simulink model "BLDCmotorControl_FOC_R2017b_fixdt"  (R2017b)
settings: Solver=FixedStepDiscrete  StartTime=0  StopTime=0.5  FixedStep=Ts  MaxStep=1e-6  RelTol=1e-6  AbsTol=1e-6  EnableMultiTasking=on
PreLoadFcn:
  | addpath(pwd);
  | addpath(genpath('01_Libraries'));
  | addpath(genpath('02_Figures'));
  | addpath(genpath('03_CreateParamTable'));
InitFcn:
  | init_model;
values from neighbouring files (symbols this model uses):
  a_elecAngle = 60    [init_model.m]
  b_diagEna = 1    [init_model.m]
  b_fieldWeakEna = 0    [init_model.m]
  b_selPhaABCurrMeas = 1    [init_model.m]
  cf_currFilt = 0.12    [init_model.m]
  cf_idKb = 1000 * Ts_ctrl    (= 0.06)    [init_model.m]
  cf_idKi = 100 * Ts_ctrl    (= 0.006)    [init_model.m]
  cf_idKp = 1    [init_model.m]
  cf_iqKb = 1000 * Ts_ctrl    (= 0.06)    [init_model.m]
  cf_iqKi = 100 * Ts_ctrl    (= 0.006)    [init_model.m]
  cf_iqKiLimProt = 40.7 * Ts_ctrl    (= 0.002442)    [init_model.m]
  cf_iqKp = 0.5    [init_model.m]
  cf_iqKpLimProt = 7.2    [init_model.m]
  cf_nKb = 1000 * Ts_ctrl    (= 0.06)    [init_model.m]
  cf_nKi = 20.4 * Ts_ctrl    (= 0.001224)    [init_model.m]
  cf_nKp = 1.18    [init_model.m]
  cf_nKpLimProt = 5    [init_model.m]
  cf_speedCoef = round(f_ctrl * a_mechAngle * (pi/180) * (30/pi))    [init_model.m]
  CTRL_COM = 0    [init_model.m]
  dV_openRate = 1000 * Ts_ctrl    (= 0.06)    [init_model.m]
  dz_cntTrnsDetHi = 40    [init_model.m]
  dz_cntTrnsDetLo = 20    [init_model.m]
  i_max = i_max * i_sca    (= 750)    [init_model.m]
  id_fieldWeak_M1 = [  0   0  0.05  0.25    1    2    3    4  4.5  4.8   5   5] * i_sca    [init_model.m]
  iq_max_M1 = sqrt(i_max^2 - iq_max_XA.^2)    [init_model.m]
  n_commAcvLo = 15    [init_model.m]
  n_commDeacvHi = 30    [init_model.m]
  n_max = 800    [init_model.m]
  n_stdStillDet = 3    [init_model.m]
  OPEN_MODE = 0    [init_model.m]
  r_cos_M1 = cos((a_elecAngle_XA + 30)*(pi/180))    [init_model.m]
  r_errInpTgtThres = 200    [init_model.m]
  r_sin_M1 = sin((a_elecAngle_XA + 30)*(pi/180))    [init_model.m]
  r_whl = 6.5 * 2.54 * 1e-2 / 2    (= 0.08255)    [init_model.m]
  SPD_MODE = 2    [init_model.m]
  t_errDequal = 2.0 * f_ctrl    (= 32000)    [init_model.m]
  t_errQual = 0.6 * f_ctrl    (= 9600)    [init_model.m]
  TRQ_MODE = 3    [init_model.m]
  Ts = 5e-6    (= 5e-06)    [init_model.m]
  Ts_ctrl = 6e-5    (= 6e-05)    [init_model.m]
  Vd_max = 1000 - V_margin    (= 900)    [init_model.m]
  vec_hallToPos = [0 2 0 1 4 3 5 0]    [init_model.m]
  VLT_MODE = 1    [init_model.m]
  Vq_max_M1 = sqrt(Vd_max^2 - Vq_max_XA.^2)    [init_model.m]
  z_commutMap_M1 = [-1 -1  0  1  1  0 ... (first row only)    [init_model.m]
  z_ctrlModReq = 1    [init_model.m]
  z_ctrlTypSel = 1    [init_model.m]
  z_maxCntRst = 2000    [init_model.m]
undefined symbols (not defined in the file or in its folder): DiscIntNeverNeededParam, sigbuilder_block, V_max, V_min
libraries: BLDC_controller_Lib x11, simulink x11, powerlib x6, pePwmGenerator x1
(part 1 of 3)
Description:
  | This model implements FOC controller for a BLDC motor.
  | The controller is capable for embedded code generation.
  | 
  | Copyright © 2019 Emanuel FERU
settings Model: ExtModeAutoUpdateStatusClock=off  TunableVars=Vd_max,Vq_max_M1,Vq_max_XA,b_diagEna,b_fieldWeakEna,b_selPhaABCurrMeas,cf_currFilt,cf_idKb,cf_idKi,cf_idKp,cf_iqKb,cf_iqKi,cf_iqKiLimProt,cf_iqKp,cf_iqKpLimProt,cf_nKb,cf_nKi,cf_nKp,cf_nKpLimProt,cf_speedCoef,dV_openRate,dz_cntTrnsDetHi,dz_cntTrnsDetLo,i_max,id_fieldWeak_M1,iq_max_M1,iq_max_XA,n_commAcvLo,n_commDeacvHi,n_fieldWeak_XA,n_max,n_stdStillDet,r_errInpTgtThres,t_errDequal,t_errQual,z_ctrlTypSel,z_maxCntRst  TunableVarsStorageClass=Auto,Auto,Auto,Auto,Auto,Auto,Auto,Auto,Auto,Auto,Auto,Auto,Auto,Auto,Auto,Auto,Auto,Auto,Auto,Auto,Auto,Auto,Auto,Auto,Auto,Auto,Auto,Auto,Auto,Auto,Auto,Auto,Auto,Auto,Auto,Auto,Auto  TunableVarsTypeQualifier=,,,,,,,,,,,,,,,,,,,,,,,,,,,,,,,,,,,,  Creator=MathWorks  LastModifiedBy=eferu
settings SolverCC: AutoInsertRateTranBlk=on
settings DataIOCC: LimitDataPoints=on  SaveFormat=Array  ReturnWorkspaceOutputs=on  SignalLoggingName=sigsOut
settings OptimizationCC: DefaultParameterBehavior=Inlined  UseDivisionForNetSlopeComputation=on  UseFloatMulNetSlope=on  UseSpecifiedMinMax=on  InlineInvariantSignals=on  PassReuseOutputArgsAs=Individual arguments  ExpressionDepthLimit=2147483647  ZeroExternalMemoryAtStartup=off  ZeroInternalMemoryAtStartup=off  NoFixptDivByZeroProtection=on  EfficientFloat2IntCast=on  LifeSpan=1  OptimizeBlockOrder=speed  DifferentSizesBufferReuse=on
settings DebuggingCC: ReadBeforeWriteMsg=DisableAll  WriteAfterWriteMsg=DisableAll  WriteAfterReadMsg=DisableAll  UnderspecifiedInitializationDetection=Classic  InheritedTsInSrcMsg=none  MultiTaskDSMMsg=none  MultiTaskCondExecSysMsg=none  ParameterTunabilityLossMsg=error  FcnCallInpInsideContextMsg=warning  StateNameClashWarn=warning  SFUnexpectedBacktrackingDiag=warning  SFNoUnconditionalDefaultTransitionDiag=warning  SFExecutionAtInitializationDiag=none
settings HardwareCC: ProdBitPerPointer=32  ProdBitPerSizeT=32  ProdBitPerPtrDiffT=32  ProdLargestAtomicInteger=Long  ProdLargestAtomicFloat=Double  ProdWordSize=32  ProdHWDeviceType=ARM Compatible->ARM Cortex  TargetUnknown=on
settings ModelReferenceCC: UpdateModelReferenceTargets=IfOutOfDate  PropagateSignalLabelsOutOfModel=off
settings SFSimCC: SFSimEcho=off  MATLABDynamicMemAlloc=off
settings RTWCC: SystemTargetFile=ert.tlc  GenCodeOnly=on  TemplateMakefile=ert_default_tmf  GenerateReport=on  BuildConfiguration=Faster Runs  IncludeHyperlinkInReport=on  LaunchReport=on  GenerateTraceInfo=on  GenerateTraceReport=on  GenerateTraceReportSl=on  GenerateTraceReportSf=on  GenerateTraceReportEml=on  GenerateWebview=on  GenerateCodeMetricsReport=on  GenerateCodeReplacementReport=on
settings CodeAppCC: ForceParamTrailComments=on  IgnoreCustomStorageClasses=off  OperatorAnnotations=on  SimulinkDataObjDesc=on  SFDataObjDesc=on  CustomSymbolStrGlobalVar=rt$N$M  CustomSymbolStrType=$N$M  CustomSymbolStrFcn=$N$M$F  CustomSymbolStrMacro=$N$M  InsertBlockDesc=on
settings ERTTargetCC: GenerateSampleERTMain=on  IncludeMdlTerminateFcn=off  CombineSignalStateStructs=on  SuppressErrorStatus=on  MultiInstanceERTCode=on  CodeInterfacePackaging=Reusable function  SupportNonFinite=off  SupportComplex=off  InlinedParameterPlacement=NonHierarchical  RootIOFormat=Part of model data structure  ERTCustomFileTemplate=example_file_process.tlc  ERTFilePackagingFormat=CompactWithDataFile  PreserveStaticInFcnDecls=off
settings ConfigComp: CovMetricSettings=dw  CovHtmlReporting=on  CovSaveCumulativeToWorkspaceVar=on  CovSaveSingleToWorkspaceVar=on  CovExternalEMLEnable=off  CovSFcnEnable=off
settings SimscapeCC: SimscapeNormalizeSystem=off

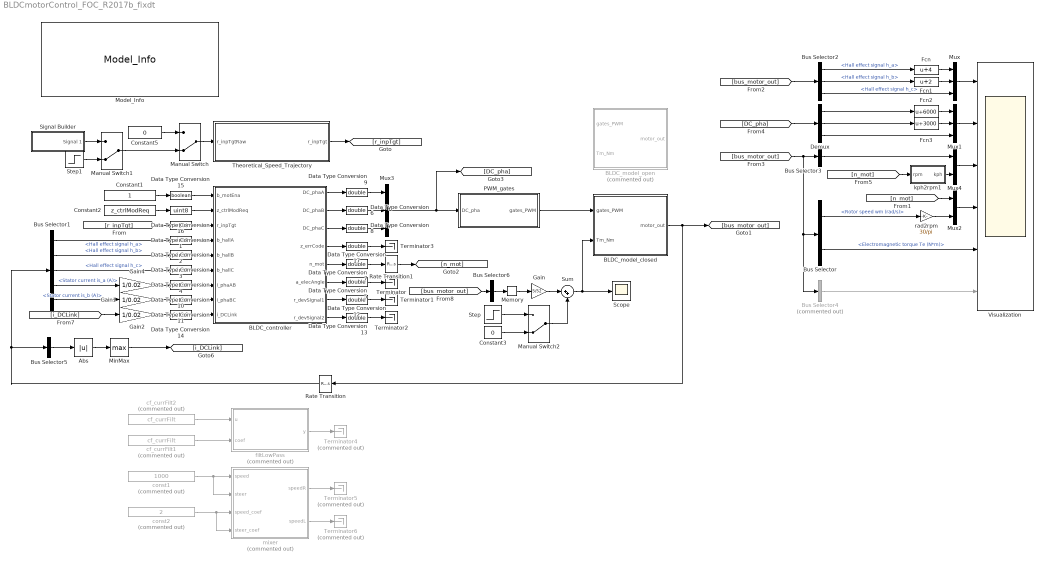
== system BLDCmotorControl_FOC_R2017b_fixdt ==
  Abs : Abs
  BLDC_controller : Subsystem  TreatAsAtomicUnit=on  SystemSampleTime=Ts_ctrl
  BLDC_model_closed : Subsystem
      mask help: Simulink:masks:GenSFuncDesc_MD
      mask Help: eval('feval(''rtwprivate'',''rtwhelpview'',''rtw_sfcn_block'')');
  BLDC_model_open : Subsystem  Commented=on
  Bus Selector : BusSelector  OutputSignals=Rotor speed wm (rad/s),Electromagnetic torque Te (N*m)
  Bus Selector1 : BusSelector  OutputSignals=Hall effect signal h_a,Hall effect signal h_b,Hall effect signal h_c,Stator current is_a (A),Stator current is_b (A)
  Bus Selector2 : BusSelector  OutputSignals=Hall effect signal h_a,Hall effect signal h_b,Hall effect signal h_c
  Bus Selector3 : BusSelector  OutputSignals=Stator current is_a (A),Stator current is_b (A),Stator current is_c (A)  OutputAsBus=on
  Bus Selector4 : BusSelector  Commented=on  OutputSignals=Stator back EMF e_a (V),Stator back EMF e_b (V),Stator back EMF e_cV)  OutputAsBus=on
  Bus Selector5 : BusSelector  OutputSignals=Stator current is_a (A),Stator current is_b (A),Stator current is_c (A)  OutputAsBus=on
  Bus Selector6 : BusSelector  OutputSignals=Rotor speed wm (rad/s)  OutputAsBus=on
  Constant1 : Constant  OutDataTypeStr=double
  Constant2 : Constant  Value=z_ctrlModReq  OutDataTypeStr=double
  Constant3 : Constant  Value=0  OutDataTypeStr=double
  Constant5 : Constant  Value=0  OutDataTypeStr=double
  Data Type Conversion{1,10..11,14} (4 alike) : DataTypeConversion  OutDataTypeStr=int16  RndMeth=Zero
  Data Type Conversion{5..9,12..13,17} (8 alike) : DataTypeConversion  OutDataTypeStr=double  RndMeth=Zero
  Data Type Conversion15 : DataTypeConversion  OutDataTypeStr=boolean  RndMeth=Zero
  Data Type Conversion{2..4,16} (4 alike) : DataTypeConversion  OutDataTypeStr=uint8  RndMeth=Zero
  Demux : Demux  Outputs=3
  Fcn : Fcn  Expr=u+4
  Fcn1 : Fcn  Expr=u+2
  Fcn2 : Fcn  Expr=u+6000
  Fcn3 : Fcn  Expr=u+3000
  Gain : Gain  Gain=5/52
  Gain1 : Gain  Tag=struct('comment',struct('text','','placement',1),'logdata',struct('maxnumvals',inf,'plotchannels',[],'loggingmode',3,'channels',1),'output',struct('variable','','description','','name','$S_$B','width',1,'address','','max',NaN,'min',NaN,'class','default','type','CONTINUOUS','scaling','','lsb',1,'offset',0,'arb',0,'freeze',1,'unit','','autoscalingmode',1,'lowerheadroom',1,'upperheadroom',1,'headroomunit','bit','keepdatatype',1,'checkmin',0,'checkmax',0,'castoutput',0,'show',0),'gain',struct('variable','','description','','name','$S_$B_gain','width',1,'address','','max',NaN,'min',NaN,'class','default','type','CONTINUOUS','scaling','','lsb',1,'offset',0,'arb',0,'freeze',1,'unit','','keepdatatype',1,'value','1','scalar',0,'tolerance',1),'scalingvalid',0,'date',730486)  Gain=1/0.02  RndMeth=Zero  SaturateOnIntegerOverflow=on  OutDataTypeStr=Inherit: Same as input  ParamDataTypeStr=Inherit: Same as input
  Gain2 : Gain  Tag=struct('comment',struct('text','','placement',1),'logdata',struct('maxnumvals',inf,'plotchannels',[],'loggingmode',3,'channels',1),'output',struct('variable','','description','','name','$S_$B','width',1,'address','','max',NaN,'min',NaN,'class','default','type','CONTINUOUS','scaling','','lsb',1,'offset',0,'arb',0,'freeze',1,'unit','','autoscalingmode',1,'lowerheadroom',1,'upperheadroom',1,'headroomunit','bit','keepdatatype',1,'checkmin',0,'checkmax',0,'castoutput',0,'show',0),'gain',struct('variable','','description','','name','$S_$B_gain','width',1,'address','','max',NaN,'min',NaN,'class','default','type','CONTINUOUS','scaling','','lsb',1,'offset',0,'arb',0,'freeze',1,'unit','','keepdatatype',1,'value','1','scalar',0,'tolerance',1),'scalingvalid',0,'date',730486)  Gain=1/0.02  RndMeth=Zero  SaturateOnIntegerOverflow=on  OutDataTypeStr=Inherit: Same as input  ParamDataTypeStr=Inherit: Same as input
  Gain4 : Gain  Tag=struct('comment',struct('text','','placement',1),'logdata',struct('maxnumvals',inf,'plotchannels',[],'loggingmode',3,'channels',1),'output',struct('variable','','description','','name','$S_$B','width',1,'address','','max',NaN,'min',NaN,'class','default','type','CONTINUOUS','scaling','','lsb',1,'offset',0,'arb',0,'freeze',1,'unit','','autoscalingmode',1,'lowerheadroom',1,'upperheadroom',1,'headroomunit','bit','keepdatatype',1,'checkmin',0,'checkmax',0,'castoutput',0,'show',0),'gain',struct('variable','','description','','name','$S_$B_gain','width',1,'address','','max',NaN,'min',NaN,'class','default','type','CONTINUOUS','scaling','','lsb',1,'offset',0,'arb',0,'freeze',1,'unit','','keepdatatype',1,'value','1','scalar',0,'tolerance',1),'scalingvalid',0,'date',730486)  Gain=1/0.02  RndMeth=Zero  SaturateOnIntegerOverflow=on  OutDataTypeStr=Inherit: Same as input  ParamDataTypeStr=Inherit: Same as input
  Manual Switch : ManualSwitch  CurrentSetting=0
  Manual Switch1 : ManualSwitch  CurrentSetting=0
  Manual Switch2 : ManualSwitch  CurrentSetting=0
  Memory : Memory
  MinMax : MinMax  Function=max
  Model_Info : BLDC_controller_Lib/Model_Info
  Mux : Mux  Inputs=3
  Mux1 : Mux  Inputs=3
  Mux2 : Mux  Inputs=2
  Mux3 : Mux  Inputs=3
  Mux4 : Mux  Inputs=2
  PWM_gates : Subsystem
  Rate Transition : RateTransition  Integrity=off  Deterministic=off
  Rate Transition1 : RateTransition  Integrity=off  Deterministic=off
  Scope : Scope
  Signal Builder : Subsystem  Tag=STV Subsys  LoadFcn=sigbuilder_block('load');  StartFcn=sigbuilder_block('start');  StopFcn=sigbuilder_block('stop');  ClipboardFcn=sigbuilder_block('clipboard');  mask(Sigbuilder block){tuvar=[0:10]}
      mask help: Simulink:masks:SigbuilderBlock_MD
      mask init:
      | if ~strcmp(get_param(bdroot(gcbh),'SimulationStatus'),'stopped') tuvar = sigbuilder_block('maskInit'); end
      settings: CopyFcn=sigbuilder_block('copy');  DeleteFcn=sigbuilder_block('delete');  ModelCloseFcn=sigbuilder_block('modelClose');  PreSaveFcn=sigbuilder_block('preSave');  PauseFcn=sigbuilder_block('pause');  ContinueFcn=sigbuilder_block('continue');  NameChangeFcn=sigbuilder_block('namechange');  OpenFcn=sigbuilder_block('open',[141.283 165.057 550.868 400.075 ]);  CloseFcn=sigbuilder_block('close');
      mask Display: plot(0, 0, 100, 100,[2, 2, 32, 32, 2], [68, 8, 8, 68, 68],[32, 2], [38, 38], [32, 19, 2],[53, 60, 44], [32, 17, 17, 2],[16, 16, 31, 31]);txt = getActiveGroup(gcbh);text(2, 100, txt,'verticalAlignment', 'top');
  Step : Step  Time=0.25  Before=-5  After=5  SampleTime=0
  Step1 : Step  Time=0.25  Before=1000  After=-1000
  Sum : Sum  Inputs=|++
  Terminator{,1..3} (4 alike) : Terminator
      settings: Tag=Controls_Lib  Description=Terminator  CopyFcn=Lib_CopyFcn(gcb);  PreDeleteFcn=Lib_PreDeleteFcn(gcb);
  Terminator4 : Terminator  Commented=on
      settings: Tag=Controls_Lib  Description=Terminator  CopyFcn=Lib_CopyFcn(gcb);  PreDeleteFcn=Lib_PreDeleteFcn(gcb);
  Terminator5 : Terminator  Commented=on
      settings: Tag=Controls_Lib  Description=Terminator  CopyFcn=Lib_CopyFcn(gcb);  PreDeleteFcn=Lib_PreDeleteFcn(gcb);
  Terminator6 : Terminator  Commented=on
      settings: Tag=Controls_Lib  Description=Terminator  CopyFcn=Lib_CopyFcn(gcb);  PreDeleteFcn=Lib_PreDeleteFcn(gcb);
  Theoretical_Speed_Trajectory : Subsystem
  Visualization : Scope  NumInputPorts=6
  cf_currFilt1 : Constant  Commented=on  Value=cf_currFilt  OutDataTypeStr=fixdt(0,16,16)
  cf_currFilt2 : Constant  Commented=on  Value=cf_currFilt  OutDataTypeStr=int16
  const1 : Constant  Commented=on  Value=1000  OutDataTypeStr=fixdt(1,16,4)
  const2 : Constant  Commented=on  Value=2  OutDataTypeStr=fixdt(1,16,14)
  filtLowPass : Subsystem  Commented=on  TreatAsAtomicUnit=on
      settings: RTWFcnNameOpts=Use subsystem name
  kph2rpm1 : Subsystem
  mixer : Subsystem  Commented=on  TreatAsAtomicUnit=on
      settings: RTWFcnNameOpts=Use subsystem name
  rad2rpm : Gain  Gain=30/pi
  wires:
  Mux2/1 -> Visualization/4
  Bus Selector/1 -> rad2rpm/1  "<Rotor speed wm (rad/s)>"
  Bus Selector/2 -> Visualization/5  "<Electromagnetic torque Te (N*m)>"
  Bus Selector2/3 -> Mux/3  "<Hall effect signal h_c>"
  Bus Selector2/2 -> Fcn1/1  "<Hall effect signal h_b>"
  Bus Selector2/1 -> Fcn/1  "<Hall effect signal h_a>"
  Fcn1/1 -> Mux/2
  Mux/1 -> Visualization/1
  Fcn/1 -> Mux/1
  Demux/1 -> Fcn2/1
  Demux/2 -> Fcn3/1
  Fcn2/1 -> Mux1/1
  Fcn3/1 -> Mux1/2
  Demux/3 -> Mux1/3
  Mux1/1 -> Visualization/2
  Bus Selector4/1 -> Visualization/6
  rad2rpm/1 -> Mux2/2
  BLDC_controller/5(n_mot) -> Data Type Conversion7/1
  Sum/1 -> BLDC_model_closed/2(Tm_Nm), Scope/1
  Bus Selector1/2 -> Data Type Conversion3/1  "<Hall effect signal h_b>"
  Bus Selector1/1 -> Data Type Conversion2/1  "<Hall effect signal h_a>"
  Bus Selector1/3 -> Data Type Conversion4/1  "<Hall effect signal h_c>"
  Data Type Conversion2/1 -> BLDC_controller/4("b_hallA ")
  Data Type Conversion3/1 -> BLDC_controller/5(b_hallB)
  Data Type Conversion4/1 -> BLDC_controller/6(b_hallC)
  Theoretical_Speed_Trajectory/1(r_inpTgt) -> [r_inpTgt]
  [r_inpTgt] -> Data Type Conversion1/1
  Data Type Conversion1/1 -> BLDC_controller/3(r_inpTgt)
  BLDC_controller/2(DC_phaB) -> Data Type Conversion6/1
  BLDC_controller/3(DC_phaC) -> Data Type Conversion8/1
  BLDC_controller/1(DC_phaA) -> Data Type Conversion9/1
  Data Type Conversion7/1 -> Rate Transition1/1
  BLDC_controller/6(a_elecAngle) -> Data Type Conversion5/1
  Mux3/1 -> [DC_pha], PWM_gates/1(DC_pha)
  PWM_gates/1(gates_PWM) -> BLDC_model_closed/1(gates_PWM)
  Rate Transition1/1 -> [n_mot]
  [n_mot] -> Mux2/1
  [bus_motor_out] -> Bus Selector2/1
  [bus_motor_out] -> Bus Selector3/1, Bus Selector4/1, Bus Selector/1
  [DC_pha] -> Demux/1
  Manual Switch/1 -> Theoretical_Speed_Trajectory/1(r_inpTgtRaw)
  Constant5/1 -> Manual Switch/1
  Signal Builder/1(Signal 1) -> Manual Switch1/1
  Manual Switch1/1 -> Manual Switch/2
  Step1/1 -> Manual Switch1/2
  Data Type Conversion5/1 -> Terminator/1
  Data Type Conversion8/1 -> Mux3/3
  Data Type Conversion6/1 -> Mux3/2
  Data Type Conversion9/1 -> Mux3/1
  [n_mot] -> kph2rpm1/1(rpm)
  Mux4/1 -> Visualization/3
  Bus Selector3/1 -> Mux4/1
  kph2rpm1/1(kph) -> Mux4/2
  Data Type Conversion10/1 -> BLDC_controller/7(i_phaAB)
  Data Type Conversion11/1 -> BLDC_controller/8(i_phaBC)
  Gain4/1 -> Data Type Conversion10/1
  Gain1/1 -> Data Type Conversion11/1
  BLDC_controller/7(r_devSignal1) -> Data Type Conversion12/1
  Data Type Conversion13/1 -> Terminator2/1
  BLDC_controller/8(r_devSignal2) -> Data Type Conversion13/1
  Gain2/1 -> Data Type Conversion14/1
  Data Type Conversion14/1 -> BLDC_controller/9(i_DCLink)
  [i_DCLink] -> Gain2/1
  Bus Selector1/4 -> Gain4/1  "<Stator current is_a (A)>"
  Bus Selector1/5 -> Gain1/1  "<Stator current is_b (A)>"
  Data Type Conversion15/1 -> BLDC_controller/1(b_motEna)
  Constant1/1 -> Data Type Conversion15/1
  [bus_motor_out] -> Bus Selector6/1
  Bus Selector6/1 -> Memory/1
  Gain/1 -> Sum/1
  Data Type Conversion16/1 -> BLDC_controller/2(z_ctrlModReq)
  Constant2/1 -> Data Type Conversion16/1
  Rate Transition/1 -> Bus Selector1/1, Bus Selector5/1
  Memory/1 -> Gain/1
  Step/1 -> Manual Switch2/1
  Manual Switch2/1 -> Sum/2
  Constant3/1 -> Manual Switch2/2
  Data Type Conversion17/1 -> Terminator3/1
  BLDC_controller/4(z_errCode) -> Data Type Conversion17/1
  Data Type Conversion12/1 -> Terminator1/1
  Bus Selector5/1 -> Abs/1
  BLDC_model_closed/1(motor_out) -> Rate Transition/1, [bus_motor_out]
  MinMax/1 -> [i_DCLink]
  Abs/1 -> MinMax/1
  filtLowPass/1(y) -> Terminator4/1
  cf_currFilt1/1 -> filtLowPass/2(coef)
  cf_currFilt2/1 -> filtLowPass/1(u)
  mixer/1(speedR) -> Terminator5/1
  const1/1 -> mixer/2(steer), mixer/1(speed)
  const2/1 -> mixer/4(steer_coef), mixer/3(speed_coef)
  mixer/2(speedL) -> Terminator6/1

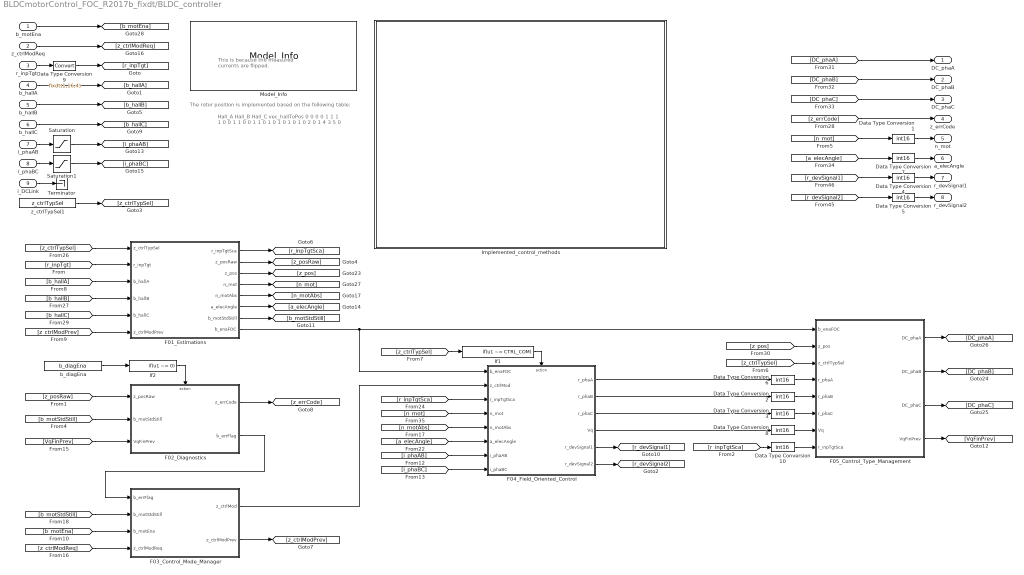
== system BLDCmotorControl_FOC_R2017b_fixdt/BLDC_controller ==
  note: The rotor position is implemented based on the following table:
  note: Hall_A
      | Hall_B
      | Hall_C
      | vec_hallToPos
      |
      | 0
      | 0
      | 0
      | 0
      | 1
      | 1
      | 1
      | 1
      | 0
      | 0
      | 1
      | 1
      | 0
      | 0
      | 1
      | 1
      | 0
      | 1
      | 0
      | 1
      | 0
      | 1
      | 0
      | 1
      | 0
      | 2
      | 0
      | 1
      | 4
      | 3
      | 5
      | 0
  note: This is because the measured currents are flipped.
  b_motEna : Inport
  z_ctrlModReq : Inport  Port=2
  r_inpTgt : Inport  Port=3
  "b_hallA " : Inport  Port=4
  b_hallB : Inport  Port=5
  b_hallC : Inport  Port=6
  i_phaAB : Inport  Port=7
  i_phaBC : Inport  Port=8
  i_DCLink : Inport  Port=9
  Data Type Conversion{1..8,10} (9 alike) : DataTypeConversion  OutDataTypeStr=int16
  Data Type Conversion9 : DataTypeConversion  OutDataTypeStr=fixdt(1,16,4)
  F01_Estimations : Subsystem
  F02_Diagnostics : Subsystem
  F03_Control_Mode_Manager : Subsystem
  F04_Field_Oriented_Control : Subsystem
  F05_Control_Type_Management : Subsystem
  If1 : If  IfExpression=u1 ~= CTRL_COM  ShowElse=off
  If2 : If  IfExpression=u1 ~= 0  ShowElse=off
  Implemented_control_methods : Subsystem
      mask Display: image('control_methods.png')
  Model_Info : BLDC_controller_Lib/Model_Info
  Saturation : Saturate  UpperLimit=1500  LowerLimit=-1500  OutDataTypeStr=fixdt(1,16,4)
  Saturation1 : Saturate  UpperLimit=1500  LowerLimit=-1500  OutDataTypeStr=fixdt(1,16,4)
  Terminator : Terminator
  b_diagEna : Constant  Value=b_diagEna  OutDataTypeStr=boolean
  z_ctrlTypSel1 : Constant  Value=z_ctrlTypSel  OutDataTypeStr=uint8
  DC_phaA : Outport
  DC_phaB : Outport  Port=2
  DC_phaC : Outport  Port=3
  z_errCode : Outport  Port=4  OutputWhenDisabled=reset  InitialOutput=0
  n_mot : Outport  Port=5
  a_elecAngle : Outport  Port=6
  r_devSignal1 : Outport  Port=7  OutputWhenDisabled=reset  InitialOutput=0
  r_devSignal2 : Outport  Port=8  OutputWhenDisabled=reset  InitialOutput=0
  wires:
  [n_mot] -> F04_Field_Oriented_Control/4(n_mot)
  F02_Diagnostics/2(b_errFlag) -> F03_Control_Mode_Manager/1(b_errFlag)
  Data Type Conversion5/1 -> r_devSignal2/1
  Data Type Conversion4/1 -> r_devSignal1/1
  If1/1 -> F04_Field_Oriented_Control/Action
  i_phaBC/1 -> Saturation1/1
  [r_devSignal1] -> Data Type Conversion4/1
  [z_ctrlTypSel] -> If1/1
  [z_pos] -> F05_Control_Type_Management/2(z_pos)
  Saturation/1 -> [i_phaAB]
  F01_Estimations/5(n_motAbs) -> [n_motAbs]
  [b_motEna] -> F03_Control_Mode_Manager/3(b_motEna)
  b_diagEna/1 -> If2/1
  Data Type Conversion10/1 -> F05_Control_Type_Management/8(r_inpTgtSca)
  [z_errCode] -> z_errCode/1
  If2/1 -> F02_Diagnostics/Action
  [n_motAbs] -> F04_Field_Oriented_Control/5(n_motAbs)
  [z_ctrlTypSel] -> F01_Estimations/1(z_ctrlTypSel)
  [DC_phaB] -> DC_phaB/1
  [z_ctrlTypSel] -> F05_Control_Type_Management/3(z_ctrlTypSel)
  [z_ctrlModReq] -> F03_Control_Mode_Manager/4(z_ctrlModReq)
  [z_posRaw] -> F02_Diagnostics/1(z_posRaw)
  Data Type Conversion1/1 -> n_mot/1
  Data Type Conversion9/1 -> [r_inpTgt]
  Data Type Conversion8/1 -> F05_Control_Type_Management/7(Vq)
  F04_Field_Oriented_Control/2(r_phaB) -> Data Type Conversion2/1
  [i_phaAB] -> F04_Field_Oriented_Control/7(i_phaAB)
  i_phaAB/1 -> Saturation/1
  Data Type Conversion6/1 -> F05_Control_Type_Management/4(r_phaA)
  F04_Field_Oriented_Control/1(r_phaA) -> Data Type Conversion6/1
  [i_phaBC] -> F04_Field_Oriented_Control/8(i_phaBC)
  [n_mot] -> Data Type Conversion1/1
  [a_elecAngle] -> Data Type Conversion7/1
  [DC_phaC] -> DC_phaC/1
  F05_Control_Type_Management/2(DC_phaB) -> [DC_phaB]
  z_ctrlModReq/1 -> [z_ctrlModReq]
  F05_Control_Type_Management/1(DC_phaA) -> [DC_phaA]
  F01_Estimations/4("n_mot ") -> [n_mot]
  F04_Field_Oriented_Control/3("r_phaC ") -> Data Type Conversion3/1
  F04_Field_Oriented_Control/6(r_devSignal2) -> [r_devSignal2]
  F01_Estimations/6(a_elecAngle) -> [a_elecAngle]
  [b_hallB] -> F01_Estimations/4(b_hallB)
  i_DCLink/1 -> Terminator/1
  F04_Field_Oriented_Control/5(r_devSignal1) -> [r_devSignal1]
  Data Type Conversion7/1 -> a_elecAngle/1
  F05_Control_Type_Management/3("DC_phaC ") -> [DC_phaC]
  Saturation1/1 -> [i_phaBC]
  b_hallB/1 -> [b_hallB]
  Data Type Conversion2/1 -> F05_Control_Type_Management/5(r_phaB)
  F01_Estimations/8(b_enaFOC) -> F05_Control_Type_Management/1(b_enaFOC), F04_Field_Oriented_Control/1(b_enaFOC)
  F02_Diagnostics/1("z_errCode ") -> [z_errCode]
  Data Type Conversion3/1 -> F05_Control_Type_Management/6(r_phaC)
  b_motEna/1 -> [b_motEna]
  b_hallC/1 -> [b_hallC]
  [a_elecAngle] -> F04_Field_Oriented_Control/6(a_elecAngle)
  [DC_phaA] -> DC_phaA/1
  F01_Estimations/2(z_posRaw) -> [z_posRaw]
  r_inpTgt/1 -> Data Type Conversion9/1
  F03_Control_Mode_Manager/1(z_ctrlMod) -> F04_Field_Oriented_Control/2(z_ctrlMod)
  [b_hallA] -> F01_Estimations/3(b_hallA)
  [r_devSignal2] -> Data Type Conversion5/1
  "b_hallA "/1 -> [b_hallA]
  F01_Estimations/3(z_pos) -> [z_pos]
  z_ctrlTypSel1/1 -> [z_ctrlTypSel]
  [b_hallC] -> F01_Estimations/5(b_hallC)
  [r_inpTgt] -> F01_Estimations/2(r_inpTgt)
  [r_inpTgtSca] -> F04_Field_Oriented_Control/3(r_inpTgtSca)
  [r_inpTgtSca] -> Data Type Conversion10/1
  F01_Estimations/1(r_inpTgtSca) -> [r_inpTgtSca]
  F03_Control_Mode_Manager/2(z_ctrlModPrev) -> [z_ctrlModPrev]
  [z_ctrlModPrev] -> F01_Estimations/6(z_ctrlModPrev)
  [b_motStdStill] -> F02_Diagnostics/2(b_motStdStill)
  [b_motStdStill] -> F03_Control_Mode_Manager/2(b_motStdStill)
  F01_Estimations/7(b_motStdStill) -> [b_motStdStill]
  [VqFinPrev] -> F02_Diagnostics/3(VqFinPrev)
  F04_Field_Oriented_Control/4(Vq) -> Data Type Conversion8/1
  F05_Control_Type_Management/4(VqFinPrev) -> [VqFinPrev]

== system BLDCmotorControl_FOC_R2017b_fixdt/BLDC_model_closed ==
  gates_PWM : Inport
  Tm_Nm : Inport  Port=2
  BLDC_model_sfcn : S-Function  FunctionName=BLDC_model_sf  SFunctionModules=""  SFunctionDeploymentMode=off  EnableBusSupport=off  SFcnStateName=DWORK0  mask{rtw_sf_name=BLDC_model_sf, showVar=off}
      mask prompts: rtw_sf_name "Simulink:masks:GenSFuncName_MP"; showVar "Simulink:masks:GenSFuncShowModuleList_MP"
      mask help: Simulink:masks:GenSFuncDesc_MD
      mask init:
      | displist = '';
      | if ~strcmp(get_param(gcb, 'FunctionName'), rtw_sf_name);
      |   set_param(gcb, 'FunctionName', rtw_sf_name);
      | end
      | % Check if we are generating code
      | rtw_mode = false;
      | if strcmpi(get_param(bdroot(gcb),'SimulationStatus'),'Initializing')
      | 	rtw_mode = strcmpi(get_param(bdroot(gcb),'BuildingRTWCode'),'on') && ...
      | 		~strcmpi(get_param(bdroot(gcb),'TargetStyle'),'SimulationTarget');
      | end
      | if showVar || rtw_mode
      | 	if exist('rtwsfunc') == 2 | exist('rtwsfunc') == 6
      | 		tmplist = rtwsfunc(rtw_sf_name,gcb);
      | 		tmplist = DAStudio.message('Simulink:masks:GenSFuncListOfModules_IC', tmplist);
      | 	elseif showVar
      | 		tmplist1 = DAStudio.message('Simulink:masks:GenSFuncListOfModules_IC', '');
      |         tmplist2 = DAStudio.message('Simulink:masks:GenSFuncNotLicensed_IC');
      |         tmplist = [tmplist1 tmplist2];
      |  	end
      | end
      | if showVar
      |   displist = tmplist;
      | end
      settings: SFcnIsStateOwnerBlock=on
      settings: CopyFcn=|
      | if ~strcmp(get_param(gcb,'Linkstatus'),'none') && ...
      | ~strcmp(get_param(gcb,'Linkstatus'),'implicit')
      |   set_param(gcb,'LinkStatus','none');
      | end
      mask Help: eval('feval(''rtwprivate'',''rtwhelpview'',''rtw_sfcn_block'')');
      mask Display:
      | port_label('input',1,'gates_PWM');
      | port_label('input',2,'Tm_Nm');
      | port_label('output',1,'Stator current is_a (A)');
      | port_label('output',2,'Stator current is_b (A)');
      | port_label('output',3,'Stator current is_c (A)');
      | port_label('output',4,'Stator back EMF e_a (V)');
      | port_label('output',5,'Stator back EMF e_b (V)');
      | port_label('output',6,'Stator back EMF e_cV)');
      | port_label('output',7,'Hall effect signal h_a');
      | port_label('output',8,'Hall effect signal h_b');
      | port_label('output',9,'Hall effect signal h_c');
      | port_label('output',10,'Rotor speed wm (rad/s)');
      | port_label('output',11,'Rotor angle thetam (rad)');
      | port_label('output',12,'Electromagnetic torque Te (N*m)');
  __InputSSForSFun__ : Subsystem
  __OutputSSForSFun__ : Subsystem
  motor_out : Outport
  wires:
  gates_PWM/1 -> __InputSSForSFun__/1(gates_PWM)
  Tm_Nm/1 -> __InputSSForSFun__/2(Tm_Nm)
  __InputSSForSFun__/1(__UniqueOutportName__1__) -> BLDC_model_sfcn/1
  __InputSSForSFun__/2(__UniqueOutportName__2__) -> BLDC_model_sfcn/2
  BLDC_model_sfcn/1 -> __OutputSSForSFun__/1(__UniqueInportName__1__)
  BLDC_model_sfcn/2 -> __OutputSSForSFun__/2(__UniqueInportName__2__)
  BLDC_model_sfcn/3 -> __OutputSSForSFun__/3(__UniqueInportName__3__)
  BLDC_model_sfcn/4 -> __OutputSSForSFun__/4(__UniqueInportName__4__)
  BLDC_model_sfcn/5 -> __OutputSSForSFun__/5(__UniqueInportName__5__)
  BLDC_model_sfcn/6 -> __OutputSSForSFun__/6(__UniqueInportName__6__)
  BLDC_model_sfcn/7 -> __OutputSSForSFun__/7(__UniqueInportName__7__)
  BLDC_model_sfcn/8 -> __OutputSSForSFun__/8(__UniqueInportName__8__)
  BLDC_model_sfcn/9 -> __OutputSSForSFun__/9(__UniqueInportName__9__)
  BLDC_model_sfcn/10 -> __OutputSSForSFun__/10(__UniqueInportName__10__)
  BLDC_model_sfcn/11 -> __OutputSSForSFun__/11(__UniqueInportName__11__)
  BLDC_model_sfcn/12 -> __OutputSSForSFun__/12(__UniqueInportName__12__)
  __OutputSSForSFun__/1(motor_out) -> motor_out/1

== system BLDCmotorControl_FOC_R2017b_fixdt/BLDC_model_open ==
  gates_PWM : Inport
  Tm_Nm : Inport  Port=2
  Constant1 : Constant  Value=36
  Controlled Voltage Source1 : powerlib/Electrical Sources/Controlled Voltage Source  Initialize=on  Source_Type=DC  Amplitude=500  Phase=0  Frequency=0  Measurements=None
  Permanent Magnet Synchronous Machine : powerlib/Machines/Permanent Magnet Synchronous Machine  NbPhases=3  FluxDistribution=Trapezoidal  RotorType=Round  MechanicalLoad=Torque Tm  PresetModel=No  ShowDetailedParameters=on  MeasurementBus=off  Resistance=0.18  Inductance=0.000835  dqInductances=[8.5e-3, 8.5e-3]  La=0.000835  MachineConstant=Flux linkage established by magnets (V.s)  Flux=0.0142879  VoltageCst=44.8868  TorqueCst=0.42864  Flat=120  Mechanical=[0.00621417 0.000303448 15]  PolePairs=15  InitialConditions=[0,0, 0,0]  InitialConditions5ph=[0 0 0 0 0 0]  TsPowergui=0  TsBlock=-1  RefAngle=Aligned with phase A axis (original Park)
      settings: SourceProductName=Simscape Power Systems
  Universal Bridge1 : powerlib/Power Electronics/Universal Bridge  Arms=3  SnubberResistance=5000  SnubberCapacitance=inf  Device=MOSFET / Diodes  Ron=1e-3  Lon=0  ForwardVoltages="[  0  0  ]"  ForwardVoltage=0  GTOparameters=[ 10e-6 , 20e-6 ]  IGBTparameters=[ 1e-6 , 2e-6 ]  Measurements=None  Measurements_2=None  converterType=Rectifier
  Vab : Scope
  Vdc : Scope
  Voltage Measurement : powerlib/Measurements/Voltage Measurement  PhasorSimulation=off  OutputType=Complex  PSBequivalent=0
  Voltage Measurement1 : powerlib/Measurements/Voltage Measurement  PhasorSimulation=off  OutputType=Complex  PSBequivalent=0
  powergui : powerlib/powergui  Priority=2  SimulationMode=Discrete  SampleTime=Ts  frequency=60  Iterations=50  frequencyindice=0  Pbase=100e6  ErrMax=1e-4  UnitsV=kV  UnitsW=MW  buscounter=0  FunctionMessages=off  echomessages=off  EnableUseOfTLC=off  CurrentSourceSwitches=off  DisableSnubberDevices=off  DisableRonSwitches=off  DisableVfSwitches=off  DisplayEquations=off  SolverType=Tustin/Backward Euler (TBE)  Interpol=off  ExternalGateDelay=off  methode=off  Ts=0  x0status=blocks  SPID=off  SwTol=0  HookPort=off  RestoreLinks=warning  ResistiveCurrentMeasurement=off  Frange=[0:2:500]  Ylog=off  Xlog=on  ShowGrid=off  save=off  variable=ZData  structure=0  ZoomFFT=on  StartTime=0.0  cycles=1  DisplayStyle=1  fundamental=60  FreqAxis=off  MaxFrequency=1000  frequencyindicesteady=1  RmsSteady=1  display=off
  motor_out : Outport
  wires:
  Constant1/1 -> Controlled Voltage Source1/1
  Tm_Nm/1 -> Permanent Magnet Synchronous Machine/1
  gates_PWM/1 -> Universal Bridge1/1
  Voltage Measurement1/1 -> Vdc/1
  Permanent Magnet Synchronous Machine/1 -> motor_out/1
  Voltage Measurement/1 -> Vab/1
  connections:
  Voltage Measurement/LConn2 -- Permanent Magnet Synchronous Machine/LConn2 -- Universal Bridge1/LConn2
  Voltage Measurement1/LConn1 -- Controlled Voltage Source1/RConn1 -- Universal Bridge1/RConn1
  Universal Bridge1/RConn2 -- Controlled Voltage Source1/LConn1 -- Voltage Measurement1/LConn2
  Universal Bridge1/LConn3 -- Permanent Magnet Synchronous Machine/LConn3
  Universal Bridge1/LConn1 -- Permanent Magnet Synchronous Machine/LConn1 -- Voltage Measurement/LConn1

== system BLDCmotorControl_FOC_R2017b_fixdt/PWM_gates ==
  DC_pha : Inport
  Abs : Abs  OutDataTypeStr=Inherit: Inherit via back propagation  RndMeth=Zero
  Abs1 : Abs  OutDataTypeStr=Inherit: Inherit via back propagation  RndMeth=Zero
  Abs2 : Abs  OutDataTypeStr=Inherit: Inherit via back propagation  RndMeth=Zero
  Constant4 : Constant  Value=0  OutDataTypeStr=Inherit: Inherit via back propagation
  Demux : Demux  Outputs=3
  Gain8 : Gain  Gain=1/1000  OutDataTypeStr=Inherit: Inherit via back propagation  RndMeth=Zero
  MinMax : MinMax  Inputs=2  OutDataTypeStr=Inherit: Inherit via back propagation  RndMeth=Zero
  MinMax1 : MinMax  Function=max  Inputs=2  OutDataTypeStr=Inherit: Inherit via back propagation  RndMeth=Zero
  MinMax2 : MinMax  Inputs=2  OutDataTypeStr=Inherit: Inherit via back propagation  RndMeth=Zero
  MinMax3 : MinMax  Function=max  Inputs=2  OutDataTypeStr=Inherit: Inherit via back propagation  RndMeth=Zero
  MinMax4 : MinMax  Inputs=2  OutDataTypeStr=Inherit: Inherit via back propagation  RndMeth=Zero
  MinMax5 : MinMax  Function=max  Inputs=2  OutDataTypeStr=Inherit: Inherit via back propagation  RndMeth=Zero
  Mux4 : Mux  Inputs=6
  PWM_generator : pePwmGenerator/PWM Generator  Commented=on  CarrCount=Up  Tper=5e-5  Ts=5e-6
      settings: SourceProductName=The database C:\Users\37ef\AppData\Roaming\MathWorks\MATLAB\R2017b\slblocks_master.db is locked, or a table in the database is locked. (database is locked)
  PWM_generator1 : Subsystem
      mask help: Simulink:masks:GenSFuncDesc_MD
      mask Help: eval('feval(''rtwprivate'',''rtwhelpview'',''rtw_sfcn_block'')');
  PWM_generator12 : Subsystem
      mask help: Simulink:masks:GenSFuncDesc_MD
      mask Help: eval('feval(''rtwprivate'',''rtwhelpview'',''rtw_sfcn_block'')');
  PWM_generator2 : Subsystem
      mask help: Simulink:masks:GenSFuncDesc_MD
      mask Help: eval('feval(''rtwprivate'',''rtwhelpview'',''rtw_sfcn_block'')');
  PWM_generator3 : Subsystem
      mask help: Simulink:masks:GenSFuncDesc_MD
      mask Help: eval('feval(''rtwprivate'',''rtwhelpview'',''rtw_sfcn_block'')');
  PWM_generator4 : Subsystem
      mask help: Simulink:masks:GenSFuncDesc_MD
      mask Help: eval('feval(''rtwprivate'',''rtwhelpview'',''rtw_sfcn_block'')');
  PWM_generator5 : Subsystem
      mask help: Simulink:masks:GenSFuncDesc_MD
      mask Help: eval('feval(''rtwprivate'',''rtwhelpview'',''rtw_sfcn_block'')');
  signal_log6 : Subsystem
  gates_PWM : Outport
  wires:
  PWM_generator4/1(PWM) -> Mux4/5
  Abs/1 -> PWM_generator1/1(DC)
  PWM_generator12/1(PWM) -> Mux4/1
  PWM_generator5/1(PWM) -> Mux4/6
  MinMax1/1 -> PWM_generator12/1(DC)
  PWM_generator3/1(PWM) -> Mux4/4
  PWM_generator1/1(PWM) -> Mux4/2
  MinMax5/1 -> PWM_generator4/1(DC)
  PWM_generator2/1(PWM) -> Mux4/3
  Abs2/1 -> PWM_generator5/1(DC)
  MinMax3/1 -> PWM_generator2/1(DC)
  Abs1/1 -> PWM_generator3/1(DC)
  Demux/1 -> MinMax/2, MinMax1/2
  MinMax4/1 -> Abs2/1
  Constant4/1 -> MinMax1/1, MinMax4/1, MinMax5/1, MinMax2/1, MinMax3/1, MinMax/1
  MinMax2/1 -> Abs1/1
  Demux/2 -> MinMax2/2, MinMax3/2
  MinMax/1 -> Abs/1
  Demux/3 -> MinMax5/2, MinMax4/2
  DC_pha/1 -> Gain8/1
  Gain8/1 -> Demux/1
  Mux4/1 -> signal_log6/1(PWM), gates_PWM/1

== system BLDCmotorControl_FOC_R2017b_fixdt/Signal Builder ==
  Demux : Demux  Tag=STV Demux  Outputs=1
  FromWs : FromWorkspace  Tag=STV FromWs  VariableName=tuvar
      SigBuilderData=|
      | common.afterFinalStr = 'Extrapolate'
      | common.sampleTime = '-1'
      | dataSet.timeRange = [0 1.5]
      | dataSet.name = 'Group 1'
      | sbobj.Groups.Name = 'Group 1'
      | sbobj.Groups.Signals.Name = 'Signal 1'
      | sbobj.Groups.Signals.XData = [0 0.2 0.4 0.6 0.8 1.5]
      | sbobj.Groups.Signals.YData = [0 800 800 600 -800 -800]
      | sbobj.Groups.TimeRange = [0 1.5]
  Signal 1 : Outport  Tag=STV Outport
  wires:
  Demux/1 -> Signal 1/1
  FromWs/1 -> Demux/1

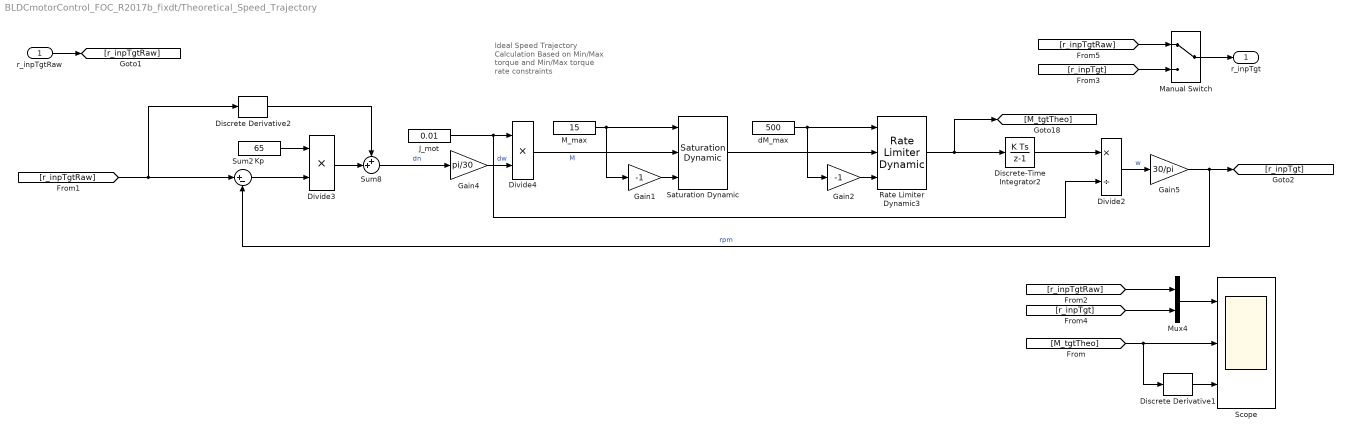
== system BLDCmotorControl_FOC_R2017b_fixdt/Theoretical_Speed_Trajectory ==
  note: Ideal Speed Trajectory Calculation
      | Based on Min/Max torque and Min/Max torque rate constraints
  r_inpTgtRaw : Inport
  Discrete Derivative1 : simulink/Discrete/Discrete Derivative  gainval=1.0  ICPrevScaledInput=0.0  OutMin=[]  OutMax=[]  OutDataType=fixdt(1, 16)  OutScaling=2^-10  DoSatur=off
  Discrete Derivative2 : simulink/Discrete/Discrete Derivative  gainval=1.0  ICPrevScaledInput=0.0  OutMin=[]  OutMax=[]  OutDataType=fixdt(1, 16)  OutScaling=2^-10  DoSatur=off
  Discrete-Time Integrator2 : DiscreteIntegrator  SampleTime=-1  ICPrevOutput=DiscIntNeverNeededParam  ICPrevScaledInput=DiscIntNeverNeededParam
  Divide2 : Product  Inputs=*/
  Divide3 : Product  Inputs=**
  Divide4 : Product  Inputs=**
  Gain1 : Gain  Gain=-1
  Gain2 : Gain  Gain=-1
  Gain4 : Gain  Gain=pi/30
  Gain5 : Gain  Gain=30/pi
  J_mot : Constant  Value=0.01  OutDataTypeStr=Inherit: Inherit via back propagation
  Kp : Constant  Value=65  OutDataTypeStr=Inherit: Inherit via back propagation
  M_max : Constant  Value=15  OutDataTypeStr=Inherit: Inherit via back propagation
  Manual Switch : ManualSwitch
  Mux4 : Mux  Inputs=2
  Rate Limiter Dynamic3 : simulink/Discontinuities/Rate Limiter Dynamic
      settings: SourceProductName=Simulink
  Saturation Dynamic : simulink/Discontinuities/Saturation Dynamic  OutMin=[]  OutMax=[]  OutDataTypeStr=Inherit: Same as second input  OutDataType=fixdt(1, 16)  OutScaling=2^-10  DoSatur=off
  Scope : Scope  NumInputPorts=3
  Sum2 : Sum  Inputs=|+-  RndMeth=Zero  OutDataTypeStr=Inherit: Same as first input
  Sum8 : Sum  Inputs=++|  RndMeth=Zero  OutDataTypeStr=Inherit: Same as first input
  dM_max : Constant  Value=500  OutDataTypeStr=Inherit: Inherit via back propagation
  r_inpTgt : Outport
  wires:
  Gain4/1 -> Divide4/2  "dw"
  M_max/1 -> Gain1/1, Saturation Dynamic/1
  J_mot/1 -> Divide2/2, Divide4/1
  Divide2/1 -> Gain5/1  "w"
  [r_inpTgtRaw] -> Discrete Derivative2/1, Sum2/1
  Divide4/1 -> Saturation Dynamic/2  "M"
  Gain1/1 -> Saturation Dynamic/3
  dM_max/1 -> Gain2/1, Rate Limiter Dynamic3/1
  Sum2/1 -> Divide3/2
  Divide3/1 -> Sum8/2
  Rate Limiter Dynamic3/1 -> [M_tgtTheo], Discrete-Time Integrator2/1
  Gain2/1 -> Rate Limiter Dynamic3/3
  Sum8/1 -> Gain4/1  "dn"
  Saturation Dynamic/1 -> Rate Limiter Dynamic3/2
  Gain5/1 -> [r_inpTgt], Sum2/2  "rpm"
  Kp/1 -> Divide3/1
  Discrete-Time Integrator2/1 -> Divide2/1
  Mux4/1 -> Scope/1
  Discrete Derivative1/1 -> Scope/3
  Discrete Derivative2/1 -> Sum8/1
  [M_tgtTheo] -> Discrete Derivative1/1, Scope/2
  r_inpTgtRaw/1 -> [r_inpTgtRaw]
  [r_inpTgtRaw] -> Mux4/1
  [r_inpTgt] -> Mux4/2
  [r_inpTgt] -> Manual Switch/2
  Manual Switch/1 -> r_inpTgt/1
  [r_inpTgtRaw] -> Manual Switch/1

== system BLDCmotorControl_FOC_R2017b_fixdt/filtLowPass ==
  u : Inport
  coef : Inport  Port=2
  Data Type Conversion : DataTypeConversion  OutDataTypeStr=fixdt(1,16,4)
  Low_Pass_Filter1 : Subsystem  TreatAsAtomicUnit=on
      settings: RTWFcnNameOpts=Use subsystem name
      mask Display:
      | plot(0,0,100,100, ...
      | [73,75,73,75,25,25,28,25,22,25],[18,20,22,20,20,84,82,84,82,84], ...
      | [25,33,33,72],[20,20,70,70],[33,34,36,39,44,50,56,66,73],[20,25,33,43,55,63,66,70,70]);
      | text(50,40,'coef'),
  y : Outport
  wires:
  coef/1 -> Low_Pass_Filter1/2(coef)
  Data Type Conversion/1 -> Low_Pass_Filter1/1(u)
  Low_Pass_Filter1/1(y) -> y/1
  u/1 -> Data Type Conversion/1

== system BLDCmotorControl_FOC_R2017b_fixdt/kph2rpm1 ==
  rpm : Inport
  Divide2 : Product  Inputs=**  RndMeth=Zero  OutDataTypeStr=Inherit: Same as first input
  Gain4 : Gain  Gain=pi/30  RndMeth=Zero  OutDataTypeStr=Inherit: Same as input
  Gain5 : Gain  Gain=3.6  RndMeth=Zero  OutDataTypeStr=Inherit: Same as input
  const2 : Constant  Value=r_whl  OutDataTypeStr=Inherit: Inherit via back propagation
  kph : Outport
  wires:
  rpm/1 -> Gain4/1
  Gain4/1 -> Divide2/1  "radps"
  const2/1 -> Divide2/2
  Divide2/1 -> Gain5/1  "mps"
  Gain5/1 -> kph/1

== system BLDCmotorControl_FOC_R2017b_fixdt/mixer ==
  speed : Inport
  steer : Inport  Port=2
  speed_coef : Inport  Port=3
  steer_coef : Inport  Port=4
  Data Type Conversion2 : DataTypeConversion  OutDataTypeStr=int16
  Data Type Conversion3 : DataTypeConversion  OutDataTypeStr=int16
  Data Type Conversion4 : DataTypeConversion  OutDataTypeStr=int16
  Display : Display
  Display1 : Display
  Display3 : Display
  Divide1 : Product  Inputs=**  RndMeth=Simplest  OutDataTypeStr=Inherit: Same as first input
  Divide2 : Product  Inputs=**  RndMeth=Simplest  OutDataTypeStr=Inherit: Same as first input
  Sum1 : Sum  Inputs=+-  RndMeth=Simplest  SaturateOnIntegerOverflow=on  InputSameDT=on  OutDataTypeStr=Inherit: Same as first input
  Sum2 : Sum  RndMeth=Simplest  SaturateOnIntegerOverflow=on  InputSameDT=on  OutDataTypeStr=Inherit: Same as first input
  speedR : Outport
  speedL : Outport  Port=2
  wires:
  Sum1/1 -> Data Type Conversion2/1
  speed/1 -> [speed]
  steer/1 -> [steer]
  speed_coef/1 -> [speed_coef]
  steer_coef/1 -> [steer_coef]
  [speed] -> Divide1/1
  [speed_coef] -> Divide1/2
  [steer] -> Divide2/1
  [steer_coef] -> Divide2/2
  Divide1/1 -> Display1/1, Data Type Conversion4/1, Sum2/1, Sum1/1
  Divide2/1 -> Sum2/2, Sum1/2
  Data Type Conversion2/1 -> speedR/1
  Data Type Conversion3/1 -> speedL/1
  Data Type Conversion4/1 -> Display/1
  Sum2/1 -> Display3/1, Data Type Conversion3/1

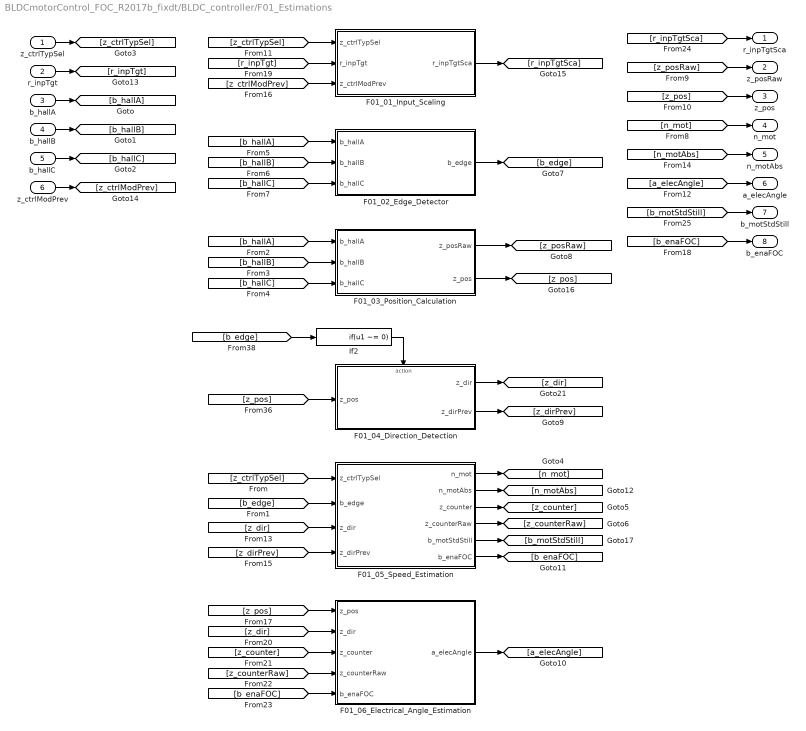
== system BLDCmotorControl_FOC_R2017b_fixdt/BLDC_controller/F01_Estimations ==
  z_ctrlTypSel : Inport
  r_inpTgt : Inport  Port=2
  b_hallA : Inport  Port=3
  b_hallB : Inport  Port=4
  b_hallC : Inport  Port=5
  z_ctrlModPrev : Inport  Port=6
  F01_01_Input_Scaling : Subsystem
  F01_02_Edge_Detector : Subsystem
  F01_03_Position_Calculation : Subsystem
  F01_04_Direction_Detection : Subsystem
  F01_05_Speed_Estimation : Subsystem
  F01_06_Electrical_Angle_Estimation : Subsystem
  If2 : If  IfExpression=u1 ~= 0  ShowElse=off
  r_inpTgtSca : Outport  OutputWhenDisabled=reset  InitialOutput=0
  z_posRaw : Outport  Port=2  OutputWhenDisabled=reset  InitialOutput=0
  z_pos : Outport  Port=3  OutputWhenDisabled=reset  InitialOutput=0
  "n_mot " : Outport  Port=4  OutputWhenDisabled=reset  InitialOutput=0
  n_motAbs : Outport  Port=5  OutputWhenDisabled=reset  InitialOutput=0
  a_elecAngle : Outport  Port=6  OutputWhenDisabled=reset  InitialOutput=0
  b_motStdStill : Outport  Port=7  OutputWhenDisabled=reset  InitialOutput=0
  b_enaFOC : Outport  Port=8
  wires:
  If2/1 -> F01_04_Direction_Detection/Action
  [b_edge] -> If2/1
  [z_pos] -> F01_04_Direction_Detection/1(z_pos)
  [b_hallA] -> F01_02_Edge_Detector/1(b_hallA)
  F01_02_Edge_Detector/1("b_edge ") -> [b_edge]
  F01_04_Direction_Detection/1(z_dir) -> [z_dir]
  [b_hallB] -> F01_02_Edge_Detector/2(b_hallB)
  [b_hallC] -> F01_02_Edge_Detector/3(b_hallC)
  b_hallA/1 -> [b_hallA]
  b_hallB/1 -> [b_hallB]
  b_hallC/1 -> [b_hallC]
  [b_hallC] -> F01_03_Position_Calculation/3(b_hallC)
  [b_hallB] -> F01_03_Position_Calculation/2(b_hallB)
  [b_hallA] -> F01_03_Position_Calculation/1(b_hallA)
  F01_03_Position_Calculation/2("z_pos ") -> [z_pos]
  [b_edge] -> F01_05_Speed_Estimation/2(b_edge)
  F01_05_Speed_Estimation/1(n_mot) -> [n_mot]
  [n_mot] -> "n_mot "/1
  [z_pos] -> z_pos/1
  [z_dir] -> F01_05_Speed_Estimation/3(z_dir)
  F01_05_Speed_Estimation/3(z_counter) -> [z_counter]
  F01_05_Speed_Estimation/4(z_counterRaw) -> [z_counterRaw]
  F01_04_Direction_Detection/2(z_dirPrev) -> [z_dirPrev]
  [z_dirPrev] -> F01_05_Speed_Estimation/4(z_dirPrev)
  [z_pos] -> F01_06_Electrical_Angle_Estimation/1(z_pos)
  [z_dir] -> F01_06_Electrical_Angle_Estimation/2(z_dir)
  [z_counter] -> F01_06_Electrical_Angle_Estimation/3(z_counter)
  [z_counterRaw] -> F01_06_Electrical_Angle_Estimation/4(z_counterRaw)
  [b_enaFOC] -> F01_06_Electrical_Angle_Estimation/5(b_enaFOC)
  F01_05_Speed_Estimation/6(b_enaFOC) -> [b_enaFOC]
  [z_ctrlTypSel] -> F01_05_Speed_Estimation/1(z_ctrlTypSel)
  [b_enaFOC] -> b_enaFOC/1
  [a_elecAngle] -> a_elecAngle/1
  F01_06_Electrical_Angle_Estimation/1(a_elecAngle) -> [a_elecAngle]
  F01_05_Speed_Estimation/2(n_motAbs) -> [n_motAbs]
  [n_motAbs] -> n_motAbs/1
  z_ctrlTypSel/1 -> [z_ctrlTypSel]
  F01_03_Position_Calculation/1(z_posRaw) -> [z_posRaw]
  [z_posRaw] -> z_posRaw/1
  [z_ctrlTypSel] -> F01_01_Input_Scaling/1(z_ctrlTypSel)
  r_inpTgt/1 -> [r_inpTgt]
  z_ctrlModPrev/1 -> [z_ctrlModPrev]
  [z_ctrlModPrev] -> F01_01_Input_Scaling/3(z_ctrlModPrev)
  [r_inpTgt] -> F01_01_Input_Scaling/2(r_inpTgt)
  [r_inpTgtSca] -> r_inpTgtSca/1
  F01_01_Input_Scaling/1(r_inpTgtSca) -> [r_inpTgtSca]
  [b_motStdStill] -> b_motStdStill/1
  F01_05_Speed_Estimation/5(b_motStdStill) -> [b_motStdStill]

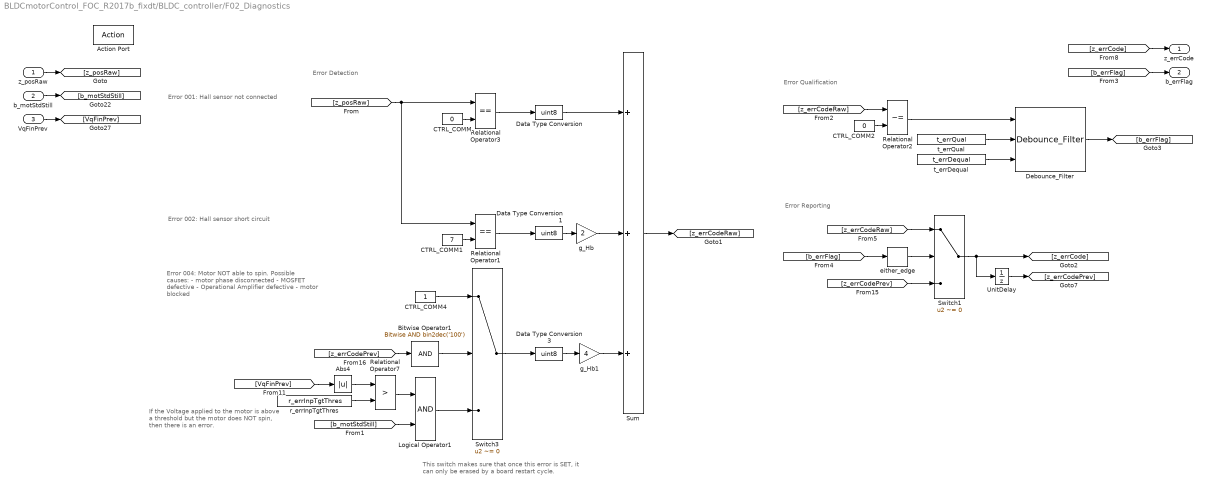
== system BLDCmotorControl_FOC_R2017b_fixdt/BLDC_controller/F02_Diagnostics ==
  note: Error 001: Hall sensor not connected
  note: Error 002: Hall sensor short circuit
  note: Error Qualification
  note: Error Detection
  note: Error Reporting
  note: Error 004: Motor NOT able to spin.
      |
      | Possible causes:
      | - motor phase disconnected
      | - MOSFET defective
      | - Operational Amplifier defective
      | - motor blocked
  note: This switch makes sure that once this error is SET, it can only be erased by a board restart cycle.
  note: If the Voltage applied to the motor is above a threshold but the motor does NOT spin, then there is an error.
  z_posRaw : Inport
  b_motStdStill : Inport  Port=2
  VqFinPrev : Inport  Port=3
  Action Port : ActionPort  InitializeStates=reset  ActionType=then
  Abs4 : Abs
  Bitwise Operator1 : simulink/Logic and Bit Operations/Bitwise Operator  logicop=AND  UseBitMask=on  BitMask=bin2dec('100')  BitMaskRealWorld=Stored Integer
  CTRL_COMM : Constant  Value=0  OutDataTypeStr=Inherit: Inherit via back propagation
  CTRL_COMM1 : Constant  Value=7  OutDataTypeStr=Inherit: Inherit via back propagation
  CTRL_COMM2 : Constant  Value=0  OutDataTypeStr=Inherit: Inherit via back propagation
  CTRL_COMM4 : Constant  OutDataTypeStr=Inherit: Inherit via back propagation
  Data Type Conversion : DataTypeConversion  OutDataTypeStr=uint8
  Data Type Conversion1 : DataTypeConversion  OutDataTypeStr=uint8
  Data Type Conversion3 : DataTypeConversion  OutDataTypeStr=uint8
  Debounce_Filter : BLDC_controller_Lib/Debounce_Filter
  Logical Operator1 : Logic  AllPortsSameDT=off  OutDataTypeStr=boolean
  Relational Operator1 : RelationalOperator  Operator===  OutDataTypeStr=boolean  RndMeth=Simplest
  Relational Operator2 : RelationalOperator  Operator=~=  OutDataTypeStr=boolean  RndMeth=Simplest
  Relational Operator3 : RelationalOperator  Operator===  OutDataTypeStr=boolean  RndMeth=Simplest
  Relational Operator7 : RelationalOperator  Operator=>  OutDataTypeStr=boolean  RndMeth=Simplest
  Sum : Sum  Inputs=+++  RndMeth=Simplest  OutDataTypeStr=Inherit: Same as first input
  Switch1 : Switch  Criteria=u2 ~= 0  OutDataTypeStr=Inherit: Inherit via back propagation  RndMeth=Zero
  Switch3 : Switch  Criteria=u2 ~= 0  OutDataTypeStr=Inherit: Inherit via back propagation  RndMeth=Zero
  UnitDelay : UnitDelay  SampleTime=-1
      settings: AttributesFormatString=Ini=%<X0>
  either_edge : BLDC_controller_Lib/either_edge
  g_Hb : Gain  Gain=2  RndMeth=Simplest  OutDataTypeStr=Inherit: Same as input
  g_Hb1 : Gain  Gain=4  RndMeth=Simplest  OutDataTypeStr=Inherit: Same as input
  r_errInpTgtThres : Constant  Value=r_errInpTgtThres  OutDataTypeStr=Inherit: Inherit via back propagation
  t_errDequal : Constant  Value=t_errDequal  OutDataTypeStr=Inherit: Inherit via back propagation
  t_errQual : Constant  Value=t_errQual  OutDataTypeStr=Inherit: Inherit via back propagation
  "z_errCode " : Outport  OutputWhenDisabled=reset  InitialOutput=0
  b_errFlag : Outport  Port=2  OutputWhenDisabled=reset  InitialOutput=0
  wires:
  [z_errCode] -> "z_errCode "/1
  z_posRaw/1 -> [z_posRaw]
  t_errDequal/1 -> Debounce_Filter/3
  t_errQual/1 -> Debounce_Filter/2
  CTRL_COMM/1 -> Relational Operator3/2
  CTRL_COMM1/1 -> Relational Operator1/2
  [z_posRaw] -> Relational Operator1/1, Relational Operator3/1
  Relational Operator3/1 -> Data Type Conversion/1
  Sum/1 -> [z_errCodeRaw]
  Relational Operator2/1 -> Debounce_Filter/1
  [z_errCodeRaw] -> Relational Operator2/1
  CTRL_COMM2/1 -> Relational Operator2/2
  Debounce_Filter/1 -> [b_errFlag]
  either_edge/1 -> Switch1/2
  Switch1/1 -> [z_errCode], UnitDelay/1
  [b_errFlag] -> b_errFlag/1
  [b_errFlag] -> either_edge/1
  [z_errCodeRaw] -> Switch1/1
  g_Hb/1 -> Sum/2
  Relational Operator1/1 -> Data Type Conversion1/1
  Data Type Conversion/1 -> Sum/1
  Data Type Conversion1/1 -> g_Hb/1
  Switch3/1 -> Data Type Conversion3/1
  Data Type Conversion3/1 -> g_Hb1/1
  g_Hb1/1 -> Sum/3
  VqFinPrev/1 -> [VqFinPrev]
  b_motStdStill/1 -> [b_motStdStill]
  [b_motStdStill] -> Logical Operator1/2
  [VqFinPrev] -> Abs4/1
  Abs4/1 -> Relational Operator7/1
  r_errInpTgtThres/1 -> Relational Operator7/2
  Relational Operator7/1 -> Logical Operator1/1
  UnitDelay/1 -> [z_errCodePrev]
  [z_errCodePrev] -> Switch1/3
  [z_errCodePrev] -> Bitwise Operator1/1
  Bitwise Operator1/1 -> Switch3/2
  CTRL_COMM4/1 -> Switch3/1
  Logical Operator1/1 -> Switch3/3

== system BLDCmotorControl_FOC_R2017b_fixdt/BLDC_controller/F03_Control_Mode_Manager ==
  b_errFlag : Inport
  b_motStdStill : Inport  Port=2
  b_motEna : Inport  Port=3
  z_ctrlModReq : Inport  Port=4
  F02_01_Mode_Transition_Calculation : Subsystem
  F02_02_Control_Mode_Manager : Stateflow chart  TreatAsAtomicUnit=on
  UnitDelay1 : UnitDelay  SampleTime=-1
  z_ctrlMod : Outport  OutputWhenDisabled=reset  InitialOutput=0
  z_ctrlModPrev : Outport  Port=2  OutputWhenDisabled=reset  InitialOutput=0
  wires:
  [z_ctrlMod] -> z_ctrlMod/1
  b_motEna/1 -> [b_motEna]
  [b_toOpen] -> F02_02_Control_Mode_Manager/1(b_toOpen)
  [b_toSpdMod] -> F02_02_Control_Mode_Manager/3(b_toSpdMod)
  z_ctrlModReq/1 -> [z_ctrlModReq]
  [b_toTrqMod] -> F02_02_Control_Mode_Manager/4(b_toTrqMod)
  UnitDelay1/1 -> [z_ctrlModPrev]
  F02_02_Control_Mode_Manager/1(z_ctrlMod) -> [z_ctrlMod], UnitDelay1/1
  [b_toActive] -> F02_02_Control_Mode_Manager/2(b_toActive)
  F02_01_Mode_Transition_Calculation/1(b_toOpen) -> [b_toOpen]
  F02_01_Mode_Transition_Calculation/2(b_toActive) -> [b_toActive]
  F02_01_Mode_Transition_Calculation/3(b_toSpdMod) -> [b_toSpdMod]
  F02_01_Mode_Transition_Calculation/4(b_toTrqMod) -> [b_toTrqMod]
  [z_ctrlModPrev] -> F02_01_Mode_Transition_Calculation/5(z_ctrlModPrev)
  [b_motEna] -> F02_01_Mode_Transition_Calculation/1(b_motEna)
  [z_ctrlModReq] -> F02_01_Mode_Transition_Calculation/4(z_ctrlModReq)
  b_errFlag/1 -> [b_errFlag]
  [b_errFlag] -> F02_01_Mode_Transition_Calculation/3(b_errFlag)
  [z_ctrlModPrev] -> z_ctrlModPrev/1
  b_motStdStill/1 -> [b_motStdStill]
  [b_motStdStill] -> F02_01_Mode_Transition_Calculation/2(b_motStdStill)
